simulink model "Single_phase_inverter"  (R2021a)
settings: Solver=VariableStepAuto  StartTime=0.0  StopTime=10.0  RelTol=1e-3
libraries: fl_lib x23, nesl_utility x16, ee_lib x14, spsRMSLib x11, spsTriangleGeneratorLib x1, spspowerguiLib x1
settings Model: Creator=Ahmed  LastModifiedBy=Ahmed
settings SolverCC: ZeroCrossAlgorithm=Adaptive
settings DebuggingCC: IgnoredZcDiagnostic=none

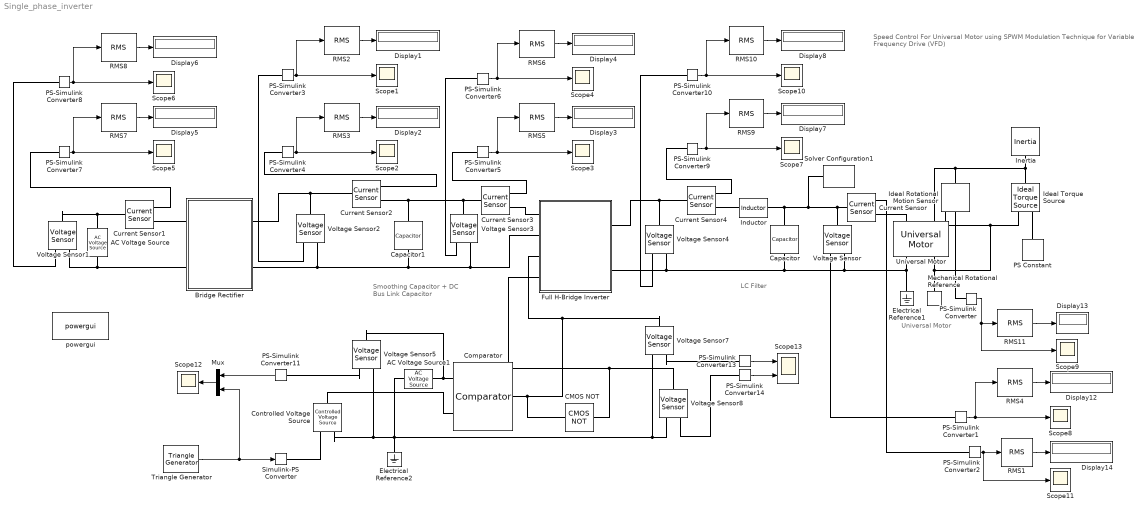
== system Single_phase_inverter ==
  note: Speed Control For Universal Motor using SPWM Modulation Technique for Variable Frequency Drive (VFD)
  note: Universal
      | Motor
  note: LC Filter
  note: Smoothing Capacitor
      | +
      | DC Bus Link Capacitor
  AC Voltage Source : fl_lib/Electrical/Electrical Sources/AC Voltage Source  amp=220*sqrt(2) V  shift=0 deg  frequency=50 Hz  omega=0 rad/s
  AC Voltage Source1 : fl_lib/Electrical/Electrical Sources/AC Voltage Source  amp=0.8 V  shift=0 deg  frequency=50 Hz  omega=0 rad/s
  Bridge Rectifier : Subsystem
  CMOS NOT : ee_lib/Integrated Circuits/Logic/CMOS NOT  V_IL=2.2 V  V_IH=5 V  C_IN=0 pF  output_type=1  V_OL=0 V  V_OH=5 V  V_CC=5 V  V_meas=5 V  R_OUT=25 Ohm  R_OH=[25, 250] Ohm  I_OH=63 mA  R_OL=[30, 800] Ohm  I_OL=-45 mA  Delay=25 ns  Ron=5 Ohm  Vf=0.6 V  output_state=1
      settings: SourceProductBaseCode=PS  InternalSimscapePortConfiguration="{\"Bottom\":[],\"Left\":[{\"id\":\"A\",\"label\":\"\",\"type\":\"foundation.electrical.electrical\"}],\"Right\":[{\"id\":\"J\",\"label\":\"\",\"type\":\"foundation.electrical.electrical\"}],\"Top\":[]}"
  Capacitor : ee_lib/Passive/Capacitor  cap_option=0  c=10 uF  Cvec=[1e-05, 1e-06] F  Vvec=[0, 10] V  CV_table_symmetry=1  f_vec=[1, 10] kHz  DFext_vec=[.8, 1.2]  C_tol=5  enable_C_tol=0  tol_distribution=1  nSigma=4  r=1e-6 Ohm  g=0 1/Ohm  averaging_period=0 s  enable_operating_limits=0  operating_limit_action=2  max_working_voltage_range=[-400, 400] V  power_rating=inf W  enable_faults=0  fault_action=1  Cscale_faulted=100  R_faulted=1e-3 Ohm  G_faulted=0 1/Ohm  tau_fault=1e-3 s  enable_temporal_fault=0  t_fault=1 s  enable_behavioral_fault=0  max_permissible_voltage_range=[-100, 100] V  t_fail_on_voltage=1 s  i_specify=off  i_priority=None  i=0 A  i_nominal_specify=off  i_nominal_unit=A  i_nominal_value=1  v_specify=off  v_priority=None  v=0 V  v_nominal_specify=off  v_nominal_unit=V  v_nominal_value=1  vc_specify=off  vc_priority=High  vc=0 V  vc_nominal_specify=off  vc_nominal_unit=V  vc_nominal_value=1
  Capacitor1 : ee_lib/Passive/Capacitor  cap_option=0  c=470 uF  Cvec=[1e-05, 1e-06] F  Vvec=[0, 10] V  CV_table_symmetry=1  f_vec=[1, 10] kHz  DFext_vec=[.8, 1.2]  C_tol=5  enable_C_tol=0  tol_distribution=1  nSigma=4  r=1e-6 Ohm  g=0 1/Ohm  averaging_period=0 s  enable_operating_limits=0  operating_limit_action=2  max_working_voltage_range=[-400, 400] V  power_rating=inf W  enable_faults=0  fault_action=1  Cscale_faulted=100  R_faulted=1e-3 Ohm  G_faulted=0 1/Ohm  tau_fault=1e-3 s  enable_temporal_fault=0  t_fault=1 s  enable_behavioral_fault=0  max_permissible_voltage_range=[-100, 100] V  t_fail_on_voltage=1 s  i_specify=off  i_priority=None  i=0 A  i_nominal_specify=off  i_nominal_unit=A  i_nominal_value=1  v_specify=off  v_priority=None  v=0 V  v_nominal_specify=off  v_nominal_unit=V  v_nominal_value=1  vc_specify=off  vc_priority=High  vc=0 V  vc_nominal_specify=off  vc_nominal_unit=V  vc_nominal_value=1
  Comparator : ee_lib/Integrated Circuits/Comparator  V_OS=0 mV  V_OL=0 V  V_OH=5 V  C_IN=0 pF  R_OUT=0 Ohm  Delay=0 s
      settings: SourceProductBaseCode=PS  InternalSimscapePortConfiguration="{\"Bottom\":[],\"Left\":[{\"id\":\"p\",\"label\":\"+\",\"type\":\"foundation.electrical.electrical\"},{\"id\":\"n\",\"label\":\"-\",\"type\":\"foundation.electrical.electrical\"}],\"Right\":[{\"id\":\"J\",\"label\":\"\",\"type\":\"foundation.electrical.electrical\"}],\"Top\":[]}"
  Controlled Voltage Source : fl_lib/Electrical/Electrical Sources/Controlled Voltage Source
  Current Sensor{,1..4} (5 alike) : fl_lib/Electrical/Electrical Sensors/Current Sensor
  Display{1..8,12..14} (11 alike) : Display
  Electrical Reference1 : fl_lib/Electrical/Electrical Elements/Electrical Reference
  Electrical Reference2 : fl_lib/Electrical/Electrical Elements/Electrical Reference
  Full H-Bridge Inverter : Subsystem
  Ideal Rotational Motion Sensor : fl_lib/Mechanical/Mechanical Sensors/Ideal Rotational Motion Sensor  wrap_angle=simscape.enum.onoff.off  offset=0 rad
  Ideal Torque Source : fl_lib/Mechanical/Mechanical Sources/Ideal Torque Source
  Inductor : ee_lib/Passive/Inductor  l=470 mH  L_tol=5  enable_L_tol=0  tol_distribution=1  nSigma=4  r=0 Ohm  g=1e-9 1/Ohm  enable_operating_limits=0  operating_limit_action=2  max_working_current=3 A  power_rating=50 W  enable_faults=0  fault_action=1  lambdaPercent=50  k_faulted=0.9999  turnsShort=0  openCct=0  groundShort=0  groundShortG=0 1/Ohm  tau_fault=1e-3 s  enable_temporal_fault=0  t_fault=1 s  enable_behavioral_fault=0  max_permissible_voltage=100 V  n_fail_on_voltage=1  max_permissible_current=1 A  t_fail_on_current=1 s  i_L_specify=off  i_L_priority=High  i_L=0 A  i_L_nominal_specify=off  i_L_nominal_unit=A  i_L_nominal_value=1
  Inertia : fl_lib/Mechanical/Rotational Elements/Inertia  inertia=2e-4 kg*m^2  num_ports=foundation.enum.numPorts2.one  w_specify=off  w_priority=High  w=0 rad/s  w_nominal_specify=off  w_nominal_unit=rad/s  w_nominal_value=1  t_specify=off  t_priority=None  t=0 N*m  t_nominal_specify=off  t_nominal_unit=N*m  t_nominal_value=1
  Mechanical Rotational Reference : fl_lib/Mechanical/Rotational Elements/Mechanical Rotational Reference
  Mux : Mux  Inputs=2
  PS Constant : fl_lib/Physical Signals/Sources/PS Constant  constant=1
  PS-Simulink Converter{,1..11,13..14} (14 alike) : nesl_utility/PS-Simulink Converter  PhysicalDomain=network_engine_domain  SubClassName=ps_output  LeftPortType=input  RightPortType=output  PseudoPeriodic=off  Frequencies=[]  Unit=inherit  AffineConversion=off
      settings: SourceProductBaseCode=PW,SS
  RMS{1..11} (11 alike) : spsRMSLib/RMS  TrueRMS=on  Freq=50  RMSInit=0  Ts=0
  Scope{1..12} (12 alike) : Scope
  Scope13 : Scope  NumInputPorts=2
  Simulink-PS Converter : nesl_utility/Simulink-PS Converter  PhysicalDomain=network_engine_domain  SubClassName=ps_input  LeftPortType=input  RightPortType=output  PseudoPeriodic=off  Frequencies=[]  NoiseDistribution=none  NoiseParameters=[]  Unit=1  AffineConversion=off  FilteringAndDerivatives=provide  SimscapeFilterOrder=1  InputFilterTimeConstant=0.001  UdotUserProvided=0
      settings: SourceProductBaseCode=PW,SS
  Solver Configuration1 : nesl_utility/Solver Configuration  PhysicalDomain=network_engine_domain  SubClassName=solver  LeftPortType=input  RightPortType=generic  Tones=[]  Harmonics=[]  SimulateNoise=off  Profile=off  UseLocalSampling=off  EnableSwitchedLinearOptims=on  FrequencyDomain=off  UseCCode=off  RelTol=0.001  AbsTol=1e-06  MinStep=1e-09  ToWorkspace=off  RevertToSquareIcSolve=off  NumHomotopyIterations=100  PhasorMode=off  PhasorModeNumHarmonics=1  DoDC=off  ResidualTolerance=1e-09  UseLocalSolver=off  LocalSolverChoice=NE_BACKWARD_EULER_ADVANCER  LocalSolverSampleTime=0.001  DoFixedCost=off  MaxNonlinIter=3  MaxModeIter=2  ComputeImpulses=off  ImpulseIterations=2  LinearAlgebra=auto  EquationFormulation=NE_TIME_EF  DelaysMemoryBudget=1024  AutomaticFiltering=on  FilteringTimeConstant=0.001  PartitionStorageMethod=AS_NEEDED  PartitionMemoryBudget=1024  PartitionMethod=ROBUST
      settings: SourceProductBaseCode=PW,SS
  Triangle Generator : spsTriangleGeneratorLib/Triangle Generator  Freq=5000  Phase=0  Ts=0
  Universal Motor : ee_lib/Electromechanical/Brushed Motors/Universal Motor  parameterization=4  Ra=132.8 Ohm  Laf=0.1722 s*V/rad/A  w_rated=1300 rpm  P_rated=16 W  V_dc=200 V  T_max=0.39 N*m  P_in=65 W  V_ac=230 V  I_ac=0.45 A  w_ac=50 Hz  Ltot=0.525 H  J=2e-4 kg*m^2  lam=1e-6 N*m/(rad/s)  speed0=0 rpm  resistance_ratio=1  alpha=[.00393, .00393] 1/K  Tmeas=25 degC  thermal_masses=[100, 100] J/K  initial_temperatures=[25, 25] degC
      settings: SourceProductBaseCode=PS  InternalSimscapePortConfiguration="{\"Bottom\":[],\"Left\":[{\"id\":\"p\",\"label\":\"+\",\"type\":\"foundation.electrical.electrical\"},{\"id\":\"R\",\"label\":\"R\",\"type\":\"foundation.mechanical.rotational.rotational\"}],\"Right\":[{\"id\":\"n\",\"label\":\"-\",\"type\":\"foundation.electrical.electrical\"},{\"id\":\"C\",\"label\":\"C\",\"type\":\"foundation.mechanical.rotational.rotational\"}],\"Top\":[]}"
  Voltage Sensor{,1..5,7..8} (8 alike) : fl_lib/Electrical/Electrical Sensors/Voltage Sensor
  powergui : spspowerguiLib/powergui  Priority=1  SimulationMode=Continuous  SampleTime=50e-6  frequency=60  Iterations=50  frequencyindice=60  Pbase=100e6  ErrMax=1e-4  UnitsV=kV  UnitsW=MW  buscounter=0  FunctionMessages=off  echomessages=off  EnableUseOfTLC=off  CurrentSourceSwitches=off  DisableSnubberDevices=off  DisableRonSwitches=off  DisableVfSwitches=off  DisplayEquations=off  AutomaticDiscreteSolvers=off  SolverType=Tustin/Backward Euler (TBE)  Interpol=off  ExternalGateDelay=off  methode=off  Ts=100  x0status=blocks  SPID=on  SwTol=0  HookPort=off  NonlinearTolerance=1e-4  nMaxIteration=100  ContinueOnMaxIteration=off  RestoreLinks=warning  ResistiveCurrentMeasurement=off  Frange=[0:2:500]  Ylog=off  Xlog=on  ShowGrid=off  save=off  variable=ZData  structure=0  ZoomFFT=off  StartTime=0.0  cycles=1  DisplayStyle=1  fundamental=60  FreqAxis=off  MaxFrequency=1000  frequencyindicesteady=1  RmsSteady=1  display=off
  wires:
  RMS4/1 -> Display12/1
  PS-Simulink Converter1/1 -> RMS4/1, Scope8/1
  RMS1/1 -> Display14/1
  PS-Simulink Converter2/1 -> RMS1/1, Scope11/1
  PS-Simulink Converter/1 -> RMS11/1, Scope9/1
  RMS11/1 -> Display13/1
  RMS2/1 -> Display1/1
  PS-Simulink Converter3/1 -> RMS2/1, Scope1/1
  RMS3/1 -> Display2/1
  PS-Simulink Converter4/1 -> RMS3/1, Scope2/1
  RMS5/1 -> Display3/1
  PS-Simulink Converter5/1 -> RMS5/1, Scope3/1
  RMS6/1 -> Display4/1
  PS-Simulink Converter6/1 -> RMS6/1, Scope4/1
  RMS7/1 -> Display5/1
  PS-Simulink Converter8/1 -> RMS8/1, Scope6/1
  PS-Simulink Converter7/1 -> RMS7/1, Scope5/1
  RMS8/1 -> Display6/1
  RMS10/1 -> Display8/1
  PS-Simulink Converter9/1 -> RMS9/1, Scope7/1
  PS-Simulink Converter10/1 -> RMS10/1, Scope10/1
  RMS9/1 -> Display7/1
  PS-Simulink Converter11/1 -> Mux/1
  Triangle Generator/1 -> Mux/2, Simulink-PS Converter/1
  Mux/1 -> Scope12/1
  PS-Simulink Converter14/1 -> Scope13/2
  PS-Simulink Converter13/1 -> Scope13/1
  connections:
  Capacitor1/LConn1 -- Current Sensor3/LConn1 -- Voltage Sensor3/LConn1 -- Current Sensor2/RConn2
  Electrical Reference1/LConn1 -- Universal Motor/RConn1 -- Voltage Sensor/RConn2 -- Voltage Sensor4/RConn2 -- Full H-Bridge Inverter/RConn2 -- Capacitor/RConn1
  Voltage Sensor8/LConn1 -- CMOS NOT/RConn1 -- Full H-Bridge Inverter/LConn4
  Ideal Torque Source/LConn1 -- Inertia/LConn1 -- Universal Motor/LConn2 -- Ideal Rotational Motion Sensor/LConn1
  Ideal Torque Source/RConn2 -- Ideal Rotational Motion Sensor/RConn1 -- Universal Motor/RConn2 -- Mechanical Rotational Reference/LConn1
  Inductor/RConn1 -- Voltage Sensor/LConn1 -- Current Sensor/LConn1 -- Solver Configuration1/RConn1 -- Capacitor/LConn1
  PS-Simulink Converter2/LConn1 -- Current Sensor/RConn1
  Current Sensor/RConn2 -- Universal Motor/LConn1
  PS-Simulink Converter/LConn1 -- Ideal Rotational Motion Sensor/RConn2
  Voltage Sensor/RConn1 -- PS-Simulink Converter1/LConn1
  PS Constant/RConn1 -- Ideal Torque Source/RConn1
  Voltage Sensor1/RConn2 -- AC Voltage Source/RConn1 -- Bridge Rectifier/LConn2
  Voltage Sensor2/LConn1 -- Current Sensor2/LConn1 -- Bridge Rectifier/RConn1
  Voltage Sensor8/RConn2 -- Voltage Sensor7/RConn2 -- Controlled Voltage Source/RConn2 -- Voltage Sensor5/RConn2 -- AC Voltage Source1/RConn1 -- Electrical Reference2/LConn1
  AC Voltage Source1/LConn1 -- Voltage Sensor5/LConn1 -- Comparator/LConn1
  CMOS NOT/LConn1 -- Comparator/RConn1 -- Voltage Sensor7/LConn1 -- Full H-Bridge Inverter/LConn3
  AC Voltage Source/LConn1 -- Current Sensor1/LConn1 -- Voltage Sensor1/LConn1
  Voltage Sensor1/RConn1 -- PS-Simulink Converter8/LConn1
  Current Sensor1/RConn1 -- PS-Simulink Converter7/LConn1
  Voltage Sensor2/RConn1 -- PS-Simulink Converter3/LConn1
  Current Sensor2/RConn1 -- PS-Simulink Converter4/LConn1
  Current Sensor3/RConn1 -- PS-Simulink Converter5/LConn1
  Voltage Sensor3/RConn1 -- PS-Simulink Converter6/LConn1
  Current Sensor4/RConn2 -- Inductor/LConn1
  Current Sensor4/RConn1 -- PS-Simulink Converter9/LConn1
  Voltage Sensor4/RConn1 -- PS-Simulink Converter10/LConn1
  Voltage Sensor5/RConn1 -- PS-Simulink Converter11/LConn1
  Voltage Sensor7/RConn1 -- PS-Simulink Converter13/LConn1
  Voltage Sensor8/RConn1 -- PS-Simulink Converter14/LConn1
  Simulink-PS Converter/RConn1 -- Controlled Voltage Source/RConn1
  Controlled Voltage Source/LConn1 -- Comparator/LConn2
  Voltage Sensor4/LConn1 -- Current Sensor4/LConn1 -- Full H-Bridge Inverter/RConn1
  Current Sensor3/RConn2 -- Full H-Bridge Inverter/LConn1
  Capacitor1/RConn1 -- Bridge Rectifier/RConn2 -- Voltage Sensor2/RConn2 -- Voltage Sensor3/RConn2 -- Full H-Bridge Inverter/LConn2
  Current Sensor1/RConn2 -- Bridge Rectifier/LConn1

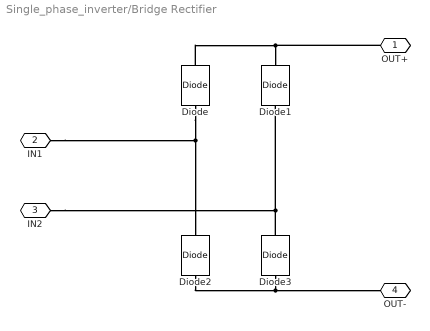
== system Single_phase_inverter/Bridge Rectifier ==
  Diode{,1..3} (4 alike) : ee_lib/Semiconductors & Converters/Diode  ModelType=ee.enum.diode.modelType.pwl  IfMat=[.07, .12, .19, 1.75, 4.24, 7.32, 11.2; .16, .3, .72, 2.14, 4.02, 6.35, 9.12] A  TjVec=[25, 125] degC  VfVec=[.5, .7, .9, 1.3, 1.7, 2.1, 2.5] V  Vf=0.6 V  Ron=0.3 Ohm  Goff=1e-8 S  prmExp=ee.enum.diode.expParam.useTwo  I12=[.0137, .545] A  V12=[.6, .7] V  IS=1e-12 A  ec=1  I1=0.0137 A  V1=0.6 V  RS=0 Ohm  Tmeas=25 degC  N_series=1  N_parallel=1  Rz=0.3 Ohm  BV=inf V  C_param=ee.enum.diode.capParam.fixed  CJ=5 pF  CJ0=5 pF  VJ=1 V  Mgrad=0.5  Vvec=[.1, 10, 100] V  Cvec=[3.5, 1, .4] pF  FC=0.5  Q_param=ee.enum.diode.recoveryParam.off  iRM=-7.15 A  iF=4 A  didt=-750 A/us  trr_factor=3  trr=115 ns  Qrr=150 s*nA  TT=50 ns  tau=100 ns  T_param=ee.enum.diode.temperatureParam.off  IS_T2=1.25e-7 A  I1_T2=0.245 A  V1_T2=0.5 V  Tmeas2=125 degC  EG_param=ee.enum.diode.egapParam.material_si  EG=1.11 eV  XTI_param=ee.enum.diode.xtiParam.pn  XTI=3  dBVdT=0 V/K  enable_faults=ee.enum.faults.faultEnable.no  fault_action=ee.enum.faults.faultAction.none  fault_types=ee.enum.diode.faults.open  tau_fault=1e-3 s  IfMat_faulted=[.07, .12, .19, 1.75, 4.24, 7.32, 11.2; .16, .3, .72, 2.14, 4.02, 6.35, 9.12] A  VfVec_faulted=[.5, .7, .9, 1.3, 1.7, 2.1, 2.5] V  Ropen_faulted=1000 Ohm  Gshort_faulted=1000 1/Ohm  Vf_faulted=0.6 V  Ron_faulted=0.3 Ohm  Goff_faulted=1e-8 S  I12_faulted=[.0137, .545] A  V12_faulted=[.6, .7] V  IS_faulted=1e-12 A  ec_faulted=1  I1_faulted=0.0137 A  V1_faulted=0.6 V  RS_faulted=0 Ohm  Rz_faulted=0.3 Ohm  BV_faulted=inf V  Cscale_faulted=100  enable_temporal_fault=ee.enum.faults.faultEnable.no  t_fault=inf s  enable_behavioral_fault=ee.enum.faults.faultEnable.no  max_permissible_voltage=inf V  n_fail_on_voltage=1  max_permissible_current=inf A  t_fail_on_current=1 s  max_permissible_dVdt=inf V/s  Tdevice=25 degC  i_specify=off  i_priority=None  i=0 A  i_nominal_specify=off  i_nominal_unit=A  i_nominal_value=1  v_specify=off  v_priority=None  v=0 V  v_nominal_specify=off  v_nominal_unit=V  v_nominal_value=1  i_diode_specify=off  i_diode_priority=None  i_diode=0 A  i_diode_nominal_specify=off  i_diode_nominal_unit=A  i_diode_nominal_value=1  v_diode_specify=off  v_diode_priority=None  v_diode=0 V  v_diode_nominal_specify=off  v_diode_nominal_unit=V  v_diode_nominal_value=1  i_capacitor_specify=off  i_capacitor_priority=None  i_capacitor=0 A  i_capacitor_nominal_specify=off  i_capacitor_nominal_unit=A  i_capacitor_nominal_value=1  v_capacitor_specify=off  v_capacitor_priority=None  v_capacitor=0 V  v_capacitor_nominal_specify=off  v_capacitor_nominal_unit=V  v_capacitor_nominal_value=1  power_dissipated_specify=off  power_dissipated_priority=None  power_dissipated=0 W  power_dissipated_nominal_specify=off  power_dissipated_nominal_unit=W  power_dissipated_nominal_value=1  max_permissible_temperature=inf K  t_fail_on_temperature=1 s  thermal_network_parameterization=ee.enum.thermalNetworkTopology.cauer  Rth=[0, 10] K/W  Rth_Foster=[4, 6] K/W  thermal_mass_parameterization=ee.enum.thermalNetwork.timeconstant  thermal_mass=[0, 1] J/K  thermal_mass_Foster=[1.5, 3] J/K  thermal_time_constant=[0, 10] s  thermal_time_constant_Foster=[6, 18] s  thermal_mass_initial_temperatures=[25, 25] degC
  OUT+ : PMIOPort  Side=Right
  IN1 : PMIOPort  Port=2  Side=Left
  IN2 : PMIOPort  Port=3  Side=Left
  OUT- : PMIOPort  Port=4  Side=Right
  connections:
  Diode2/LConn1 -- OUT-/RConn1 -- Diode3/LConn1
  OUT+/RConn1 -- Diode1/RConn1 -- Diode/RConn1
  Diode3/RConn1 -- Diode1/LConn1 -- IN2/RConn1
  Diode/LConn1 -- IN1/RConn1 -- Diode2/RConn1

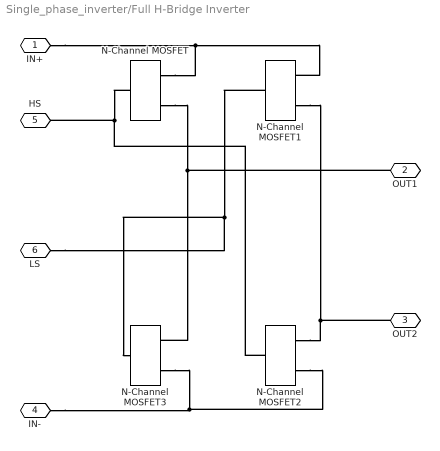
== system Single_phase_inverter/Full H-Bridge Inverter ==
  N-Channel MOSFET{,1..3} (4 alike) : ee_lib/Semiconductors & Converters/N-Channel MOSFET  paramTerminal=ee.enum.mosfet.numberOfTerminals.three  parameterization=ee.enum.mosfet.parameterization.datasheet  prmDatasheet=ee.enum.temperatureParameterization.none  prmEquCoeff=ee.enum.temperatureParameterization.none  Beta=5.0 A/V^2  Rds=0.025 Ohm  Id=6.0 A  Vgs=10 V  Vth=1.7 V  Vth0=1.7 V  lam=0 1/V  gamma_vth=0.5 V^0.50000  phib=0.5 V  Vth1=1.9071 V  Vbs1=-1 V  Vth2=2.066 V  Vbs2=-2 V  Tmeas=25 degC  RS=0.0001 Ohm  RD=0.01 Ohm  RB=0.001 Ohm  C_param=ee.enum.mosfet.capacitanceParam.fixedciss  C_GS=270 pF  C_GD=80 pF  C_DS=0 pF  C_iss=350 pF  C_rss=80 pF  C_oss=0 pF  charge_linearity_param=ee.enum.mosfet.cgdLinearity.constant  C_OX=200 pF  V_C_OX=-0.5 V  C_iss_vec=[720, 700, 590, 470, 390, 310] pF  C_rss_vec=[450, 400, 300, 190, 95, 55] pF  C_oss_vec=[900, 810, 690, 420, 270, 170] pF  C_GS_vec=[270, 300, 290, 280, 295, 255] pF  C_GD_vec=[450, 400, 300, 190, 95, 55] pF  C_DS_vec=[450, 410, 390, 230, 175, 115] pF  C_Vds_vec=[.1, .3, 1, 3, 10, 30] V  V_GS_for_cap_data=0 V  charge_linearity_param_vgb=ee.enum.mosfet.cgbLinearity.instantly  Di_param=ee.enum.mosfet.diodeParam.no  IsDiode=0 A  Vbi=0.6 V  n=1  Cj0Diode=0 pF  TT=50e-9 s  dVth_dT=-6 mV/K  dVth0_dT=-6 mV/K  Rds_T2=0.037 Ohm  Tmeas2=125 degC  BEXDatasheet=-1.5  BEXEquCoeff=-1.5  etaisDatasheet=3  etaisEquCoeff=3  Vgs_vec=[-.5, 2, 3, 4, 5] V  Vds_vec=[0, 2, 4, 8, 12, 16, 20] V  Vbs_vec=[0, -4, -6, -12] V  T_vec=[25, 125] degC  Vth_vec=[.4, 1.2, 1.4, 1.45] V  Vth_mat=[.4, .35; 1.2, 1.15; 1.4, 1.35; 1.45, 1.4] V  Ids_mat=[0, 0, 0, 0, 0, 0, 0; 0, .003, .0038, .0043, .0046, .0048, .0049; 0, .0055, .008, .009, .0095, .01, .0101; 0, .0115, .016, .018, .019, .0195, .02; 0, .0152, .0225, .0265, .028, .0295, .03] A  Ids_mat0=[0, 0, 0, 0, 0, 0, 0; 0, .003, .0038, .0043, .0046, .0048, .0049; 0, .0055, .008, .009, .0095, .01, .0101; 0, .0115, .016, .018, .019, .0195, .02; 0, .0152, .0225, .0265, .028, .0295, .03] A  Ids_mat_3D=zeros(5, 7, 2) A  Ids_mat_3D0=zeros(5, 7, 2) A  IV_table_symmetry=ee.enum.mosfet.symmetricNIV.no  VfVec=[.5, .7, .9, 1.3, 1.7, 2.1, 2.5] V  TjVec=[25, 125] degC  IfVec=[.07, .12, .19, 1.75, 4.24, 7.32, 11.2] A  IfMat=[.07, .12, .19, 1.75, 4.24, 7.32, 11.2; .16, .3, .72, 2.14, 4.02, 6.35, 9.12] A  Tmeas_dio=25 degC  etaisTabulated=3  TdeviceDatasheet=25 degC  TdeviceEquCoeff=25 degC  TdeviceTabulated=25 degC  thermal_network_parameterization=ee.enum.thermalNetworkTopology.cauer  Rth=[0, 10] K/W  Rth_Foster=[4, 6] K/W  thermal_mass_parameterization=ee.enum.thermalNetwork.timeconstant  thermal_mass=[0, 1] J/K  thermal_mass_Foster=[1.5, 3] J/K  thermal_time_constant=[0, 10] s  thermal_time_constant_Foster=[6, 18] s  thermal_mass_initial_temperatures=[25, 25] degC  betaref=18 A/V^2  Vfbref=-1.1 V  gamma=3.5 V^0.50000  phib2ref=1 V  thesatref=0.4 1/V  alpha=0  Vp=5e-2 V  thesrref=0 1/V  m=8  Tref=25 degC  Cox=1500 pF  Cgso=100 pF  Cgdo=14 pF  Rsref=2e-3 Ohm  Rdref=0.17 Ohm  Rgref=8.4 Ohm  Rbref=2e-3 Ohm  Isref=5.2e-13 A  Cj0=480 pF  Tprm=1  etabet=1.3  Stvfb=5e-4 V/K  Stphib=-8.5e-4 V/K  etasat=1.04  etasr=0.65  etar=0.95  etais=3  Tsim=25 degC  T0=[25, 25] degC
  IN+ : PMIOPort  Side=Left
  OUT1 : PMIOPort  Port=2  Side=Right
  OUT2 : PMIOPort  Port=3  Side=Right
  IN- : PMIOPort  Port=4  Side=Left
  HS : PMIOPort  Port=5  Side=Left
  LS : PMIOPort  Port=6  Side=Left
  connections:
  N-Channel MOSFET/RConn1 -- IN+/RConn1 -- N-Channel MOSFET1/RConn1
  N-Channel MOSFET/RConn2 -- OUT1/RConn1 -- N-Channel MOSFET3/RConn1
  N-Channel MOSFET/LConn1 -- N-Channel MOSFET2/LConn1 -- HS/RConn1
  N-Channel MOSFET2/RConn2 -- IN-/RConn1 -- N-Channel MOSFET3/RConn2
  N-Channel MOSFET2/RConn1 -- OUT2/RConn1 -- N-Channel MOSFET1/RConn2
  N-Channel MOSFET1/LConn1 -- LS/RConn1 -- N-Channel MOSFET3/LConn1
